simulink model "upravljani_nelinearni_i_linearni_model"  (R2015a)
settings: Solver=ode4  StartTime=0.0  StopTime=400  FixedStep=0.01  RelTol=1e-3
values from neighbouring files (symbols this model uses):
  a1 = K_dek(1, 1)    [skript_drugi_deo.m]
  a2 = K_dek(1, 2)    [skript_drugi_deo.m]
  a3 = K_dek(2, 1)    [skript_drugi_deo.m]
  a4 = K_dek(2, 2)    [skript_drugi_deo.m]
  Ar1 = 0.04    [skript_drugi_deo.m]
  Ar2 = 0.04    [skript_drugi_deo.m]
  Cd1 = 0.65    [skript_drugi_deo.m]
  Cd2 = 0.65    [skript_drugi_deo.m]
  Cdh = 0.65    [skript_drugi_deo.m]
  df1_H1 = double(subs(df1_H1, [Uvh Uv2 H1 H2], [Uvh_N Uv2_N H1_N H2_N]))    [skript_drugi_deo.m]
  df1_Uvh = double(subs(df1_Uvh, [Uvh Uv2 H1 H2], [Uvh_N Uv2_N H1_N H2_N]))    [skript_drugi_deo.m]
  df2_H1 = double(subs(df2_H1, [Uvh Uv2 H1 H2], [Uvh_N Uv2_N H1_N H2_N]))    [skript_drugi_deo.m]
  df2_H2 = double(subs(df2_H2, [Uvh Uv2 H1 H2], [Uvh_N Uv2_N H1_N H2_N]))    [skript_drugi_deo.m]
  df2_Uv2 = double(subs(df2_Uv2, [Uvh Uv2 H1 H2], [Uvh_N Uv2_N H1_N H2_N]))    [skript_drugi_deo.m]
  g = 9.81    [skript_drugi_deo.m]
  H1_max = 1.5    [skript_drugi_deo.m]
  H1_min = 0    [skript_drugi_deo.m]
  H1_N = 0.7    [skript_drugi_deo.m]
  H2_max = 1.5    [skript_drugi_deo.m]
  H2_min = 0    [skript_drugi_deo.m]
  H2_N = 0.8    [skript_drugi_deo.m]
  Kv1 = 1.5/1000    (= 0.0015)    [skript_drugi_deo.m]
  Kv2 = 1.5/1000    (= 0.0015)    [skript_drugi_deo.m]
  Kvh = 1/1000    (= 0.001)    [skript_drugi_deo.m]
  Ph = 3.25*10^5    (= 325000)    [skript_drugi_deo.m]
  ro = 1000    [skript_drugi_deo.m]
  Uv1 = 3    [skript_drugi_deo.m]
  Uv2_max = 10    [skript_drugi_deo.m]
  Uv2_min = 0    [skript_drugi_deo.m]
  Uv2_N = double(solve(e2 == 0, U2_N))    [skript_drugi_deo.m]
  Uvh_max = 10    [skript_drugi_deo.m]
  Uvh_min = 0    [skript_drugi_deo.m]
  Uvh_N = double(solve(e1 == 0, Uh_N))    [skript_drugi_deo.m]
  w1 = 0.1    [skript_drugi_deo.m]
  w2 = 0.1    [skript_drugi_deo.m]
  wh = 0.03    [skript_drugi_deo.m]
libraries: simulink x4
settings Model: Creator=Nikola  LastModifiedBy=Nikola

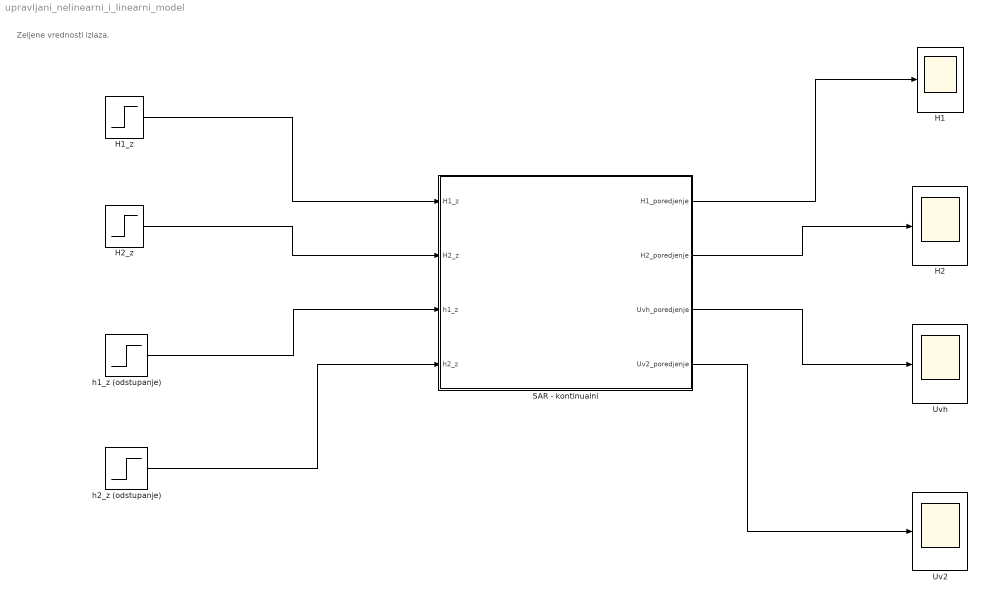
== system upravljani_nelinearni_i_linearni_model ==
  note: Zeljene vrednosti izlaza.
  " H2 " : Scope
      settings: SaveName=ScopeData4
  H1 : Scope
      settings: SaveName=ScopeData3
  "H1_z " : Step  Time=0  After=H1_N  SampleTime=0
  H2_z : Step  Time=0  After=H2_N  SampleTime=0
  SAR - kontinualni : Subsystem
  Uv2 : Scope
  "Uvh " : Scope
  h1_z (odstupanje) : Step  Time=0  After=0.1  SampleTime=0
  h2_z (odstupanje) : Step  Time=0  After=0  SampleTime=0
  wires:
  "H1_z "/1 -> SAR - kontinualni/1(H1_z)
  H2_z/1 -> SAR - kontinualni/2(H2_z)
  h1_z (odstupanje)/1 -> SAR - kontinualni/3(h1_z)
  h2_z (odstupanje)/1 -> SAR - kontinualni/4(h2_z)
  SAR - kontinualni/1(H1_poredjenje) -> H1/1
  SAR - kontinualni/2(H2_poredjenje) -> " H2 "/1
  SAR - kontinualni/3(Uvh_poredjenje) -> "Uvh "/1
  SAR - kontinualni/4(Uv2_poredjenje) -> Uv2/1

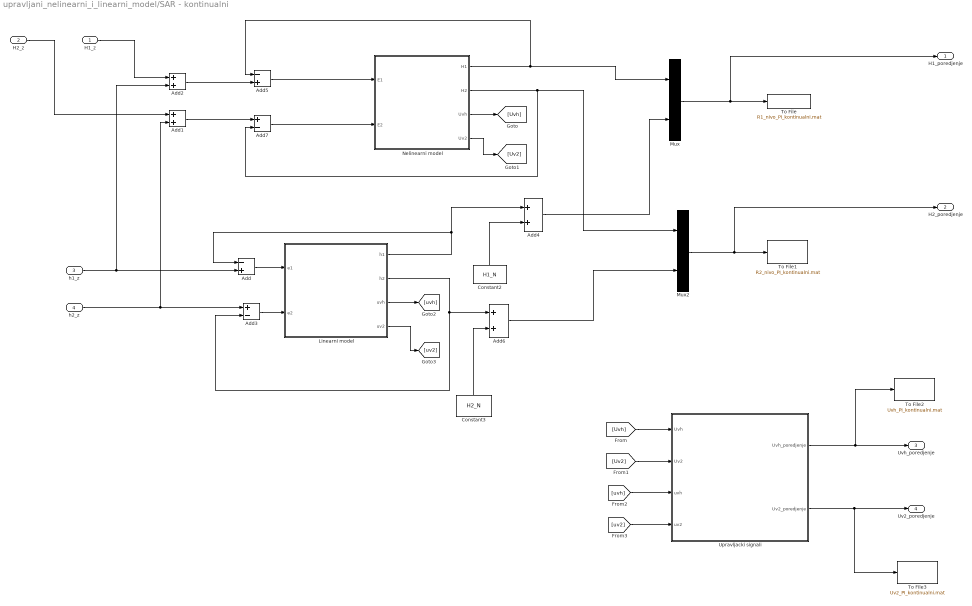
== system upravljani_nelinearni_i_linearni_model/SAR - kontinualni ==
  H1_z : Inport
  H2_z : Inport  Port=2
  h1_z : Inport  Port=3
  h2_z : Inport  Port=4
  Add : Sum  Inputs=-+
  Add{1..2,4,6} (4 alike) : Sum
  Add3 : Sum  Inputs=+-
  Add5 : Sum  Inputs=-+
  Add7 : Sum  Inputs=+-
  Constant2 : Constant  Value=H1_N
  Constant3 : Constant  Value=H2_N
  "Linearni model " : Subsystem
  Mux : Mux  Inputs=2
  Mux2 : Mux  Inputs=2
  "Nelinearni model " : Subsystem
  To File : ToFile  Filename=R1_nivo_PI_kontinualni.mat  MatrixName=H1_PI_kont
  To File1 : ToFile  Filename=R2_nivo_PI_kontinualni.mat  MatrixName=H2_PI_kont
  To File2 : ToFile  Filename=Uvh_PI_kontinualni.mat  MatrixName=Uvh_PI_kont
  To File3 : ToFile  Filename=Uv2_PI_kontinualni.mat  MatrixName=Uv2_PI_kont
  Upravljacki signali : Subsystem
  H1_poredjenje : Outport
  H2_poredjenje : Outport  Port=2
  Uvh_poredjenje : Outport  Port=3
  Uv2_poredjenje : Outport  Port=4
  wires:
  Mux/1 -> H1_poredjenje/1, To File/1
  Mux2/1 -> H2_poredjenje/1, To File1/1
  h1_z/1 -> Add2/2, Add/2
  h2_z/1 -> Add1/2, Add3/1
  Add4/1 -> Mux/2
  Add6/1 -> Mux2/2
  Constant3/1 -> Add6/2
  "Linearni model "/1(h1) -> Add4/1, Add/1
  "Linearni model "/2(h2) -> Add3/2, Add6/1
  Add/1 -> "Linearni model "/1(e1)
  Add3/1 -> "Linearni model "/2(e2)
  "Nelinearni model "/1(H1) -> Mux/1, Add5/1
  "Nelinearni model "/2(H2) -> Add7/2, Mux2/1
  Add2/1 -> Add5/2
  Add5/1 -> "Nelinearni model "/1(E1)
  Add7/1 -> "Nelinearni model "/2(E2)
  Add1/1 -> Add7/1
  Constant2/1 -> Add4/2
  "Nelinearni model "/3(Uvh) -> [Uvh]
  "Nelinearni model "/4(Uv2) -> [Uv2]
  "Linearni model "/3(uvh) -> [uvh]
  "Linearni model "/4(uv2) -> [uv2]
  H1_z/1 -> Add2/1
  H2_z/1 -> Add1/1
  [Uvh] -> Upravljacki signali/1(Uvh)
  [Uv2] -> Upravljacki signali/2(Uv2)
  Upravljacki signali/1(Uvh_poredjenje) -> To File2/1, Uvh_poredjenje/1
  Upravljacki signali/2(Uv2_poredjenje) -> To File3/1, Uv2_poredjenje/1
  [uvh] -> Upravljacki signali/3(uvh)
  [uv2] -> Upravljacki signali/4(uv2)

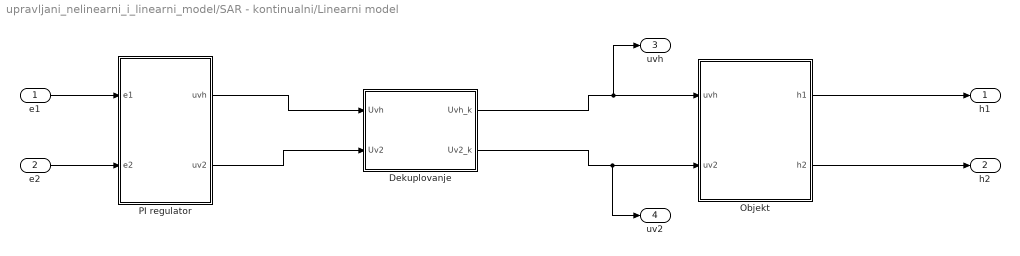
== system upravljani_nelinearni_i_linearni_model/SAR - kontinualni/Linearni model  ==
  e1 : Inport
  e2 : Inport  Port=2
  Dekuplovanje : Subsystem
  Objekt : Subsystem
  PI regulator : Subsystem
  h1 : Outport
  h2 : Outport  Port=2
  uvh : Outport  Port=3
  uv2 : Outport  Port=4
  wires:
  Objekt/1(h1) -> h1/1
  Objekt/2(h2) -> h2/1
  e1/1 -> PI regulator/1(e1)
  e2/1 -> PI regulator/2(e2)
  PI regulator/1(uvh) -> Dekuplovanje/1(Uvh)
  PI regulator/2(uv2) -> Dekuplovanje/2(Uv2)
  Dekuplovanje/1(Uvh_k) -> uvh/1, Objekt/1(uvh)
  Dekuplovanje/2(Uv2_k) -> uv2/1, Objekt/2(uv2)

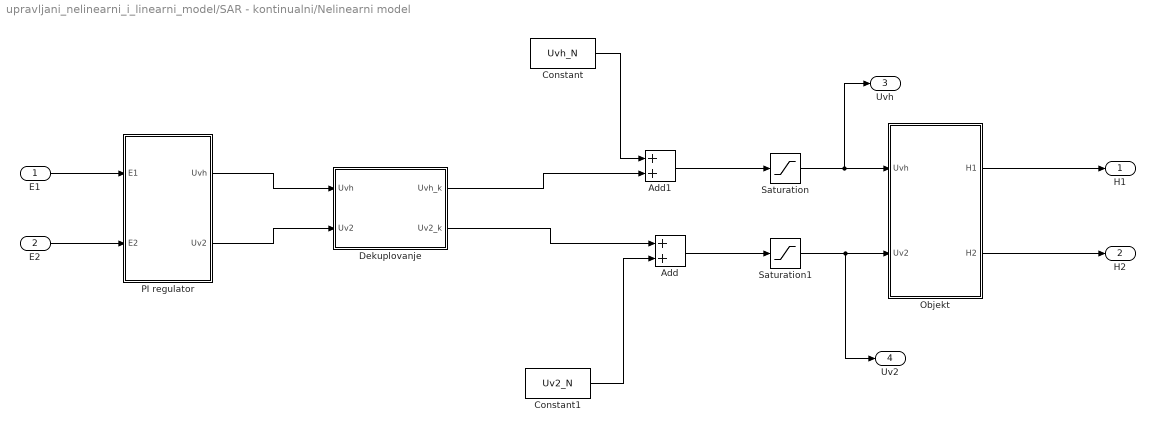
== system upravljani_nelinearni_i_linearni_model/SAR - kontinualni/Nelinearni model  ==
  E1 : Inport
  E2 : Inport  Port=2
  Add : Sum
  Add1 : Sum
  Constant : Constant  Value=Uvh_N
  Constant1 : Constant  Value=Uv2_N
  Dekuplovanje : Subsystem
  Objekt : Subsystem
  PI regulator : Subsystem
  Saturation : Saturate  UpperLimit=Uvh_max  LowerLimit=Uvh_min
  Saturation1 : Saturate  UpperLimit=Uv2_max  LowerLimit=Uv2_min
  H1 : Outport
  H2 : Outport  Port=2
  Uvh : Outport  Port=3
  Uv2 : Outport  Port=4
  wires:
  Objekt/1(H1) -> H1/1
  Objekt/2(H2) -> H2/1
  E2/1 -> PI regulator/2(E2)
  E1/1 -> PI regulator/1(E1)
  Saturation/1 -> Uvh/1, Objekt/1(Uvh)
  Saturation1/1 -> Uv2/1, Objekt/2(Uv2)
  Add1/1 -> Saturation/1
  Add/1 -> Saturation1/1
  Constant1/1 -> Add/2
  Constant/1 -> Add1/1
  Dekuplovanje/1(Uvh_k) -> Add1/2
  Dekuplovanje/2(Uv2_k) -> Add/1
  PI regulator/1(Uvh) -> Dekuplovanje/1(Uvh)
  PI regulator/2(Uv2) -> Dekuplovanje/2(Uv2)

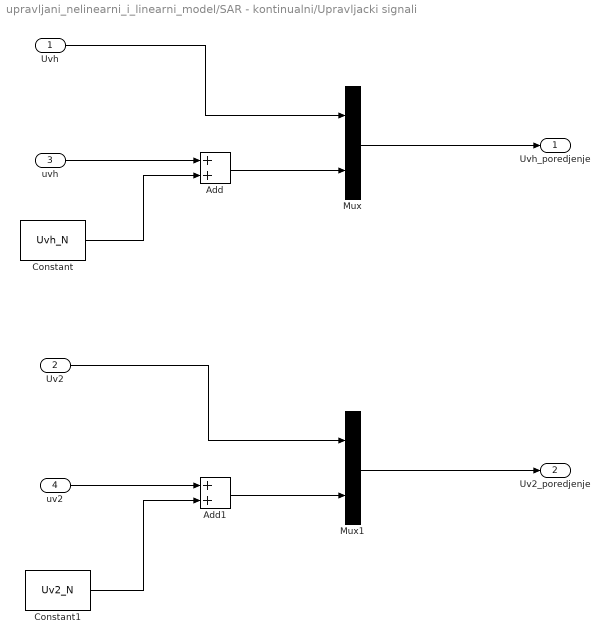
== system upravljani_nelinearni_i_linearni_model/SAR - kontinualni/Upravljacki signali ==
  Uvh : Inport
  Uv2 : Inport  Port=2
  uvh : Inport  Port=3
  uv2 : Inport  Port=4
  Add : Sum
  Add1 : Sum
  Constant : Constant  Value=Uvh_N
  Constant1 : Constant  Value=Uv2_N
  Mux : Mux  Inputs=2
  Mux1 : Mux  Inputs=2
  Uvh_poredjenje : Outport
  Uv2_poredjenje : Outport  Port=2
  wires:
  uvh/1 -> Add/1
  Constant/1 -> Add/2
  uv2/1 -> Add1/1
  Constant1/1 -> Add1/2
  Add/1 -> Mux/2
  Uvh/1 -> Mux/1
  Add1/1 -> Mux1/2
  Uv2/1 -> Mux1/1
  Mux/1 -> Uvh_poredjenje/1
  Mux1/1 -> Uv2_poredjenje/1

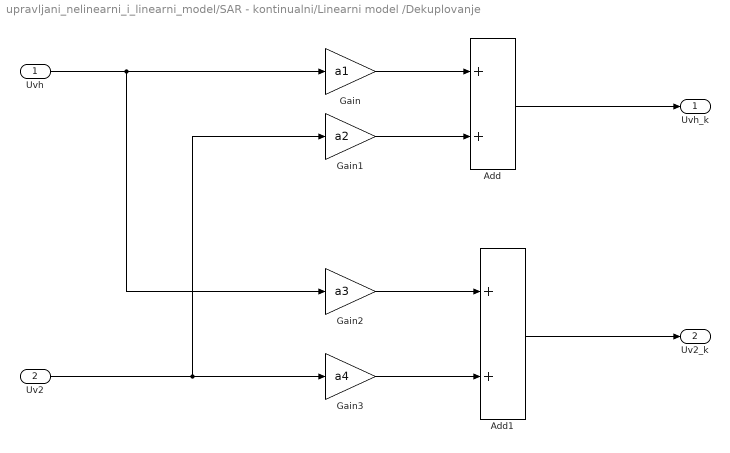
== system upravljani_nelinearni_i_linearni_model/SAR - kontinualni/Linearni model /Dekuplovanje ==
  Uvh : Inport
  Uv2 : Inport  Port=2
  Add : Sum
  Add1 : Sum
  Gain : Gain  Gain=a1
  Gain1 : Gain  Gain=a2
  Gain2 : Gain  Gain=a3
  Gain3 : Gain  Gain=a4
  Uvh_k : Outport
  Uv2_k : Outport  Port=2
  wires:
  Uvh/1 -> Gain2/1, Gain/1
  Uv2/1 -> Gain1/1, Gain3/1
  Gain/1 -> Add/1
  Gain1/1 -> Add/2
  Gain2/1 -> Add1/1
  Gain3/1 -> Add1/2
  Add/1 -> Uvh_k/1
  Add1/1 -> Uv2_k/1

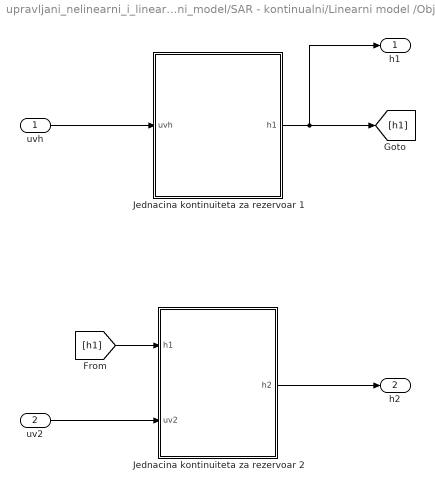
== system upravljani_nelinearni_i_linearni_model/SAR - kontinualni/Linearni model /Objekt ==
  uvh : Inport
  uv2 : Inport  Port=2
  Jednacina kontinuiteta za rezervoar 1 : Subsystem
  Jednacina kontinuiteta za rezervoar 2 : Subsystem
  h1 : Outport
  h2 : Outport  Port=2
  wires:
  Jednacina kontinuiteta za rezervoar 1/1(h1) -> [h1], h1/1
  [h1] -> Jednacina kontinuiteta za rezervoar 2/1(h1)
  Jednacina kontinuiteta za rezervoar 2/1(h2) -> h2/1
  uvh/1 -> Jednacina kontinuiteta za rezervoar 1/1(uvh)
  uv2/1 -> Jednacina kontinuiteta za rezervoar 2/2(uv2)

== system upravljani_nelinearni_i_linearni_model/SAR - kontinualni/Linearni model /PI regulator ==
  e1 : Inport
  e2 : Inport  Port=2
  PID Controller : simulink/Continuous/PID Controller  Controller=PI  TimeDomain=Continuous-time  SampleTime=-1  IntegratorMethod=Forward Euler  FilterMethod=Forward Euler  Form=Parallel  UseFilter=on  ControllerParametersSource=internal  P=6.58388823392313  I=0.318107260315565  D=0  N=100  InitialConditionSource=internal  InitialConditionForIntegrator=0  InitialConditionForFilter=0  ExternalReset=none  LimitOutput=off  UpperSaturationLimit=inf  LowerSaturationLimit=-inf  LinearizeAsGain=on  AntiWindupMode=none  Kb=1  TrackingMode=off  Kt=1  PParamMin=[]  PParamMax=[]  IParamMin=[]  IParamMax=[]  DParamMin=[]  DParamMax=[]  NParamMin=[]  NParamMax=[]  KbParamMin=[]  KbParamMax=[]  KtParamMin=[]  KtParamMax=[]  POutMin=[]  POutMax=[]  IOutMin=[]  IOutMax=[]  DOutMin=[]  DOutMax=[]  NOutMin=[]  NOutMax=[]  KbOutMin=[]  KbOutMax=[]  KtOutMin=[]  KtOutMax=[]  IntegratorOutMin=[]  IntegratorOutMax=[]  FilterOutMin=[]  FilterOutMax=[]  SumOutMin=[]  SumOutMax=[]  SumI1OutMin=[]  SumI1OutMax=[]  SumI2OutMin=[]  SumI2OutMax=[]  SumI3OutMin=[]  SumI3OutMax=[]  SumDOutMin=[]  SumDOutMax=[]  SaturationOutMin=[]  SaturationOutMax=[]  IntegratorContinuousStateAttributes=''  IntegratorStateMustResolveToSignalObject=off  IntegratorRTWStateStorageClass=Auto  FilterContinuousStateAttributes=''  FilterStateMustResolveToSignalObject=off  FilterRTWStateStorageClass=Auto  DifferentiatorICPrevScaledInput=0  DifferentiatorOutMin=[]  DifferentiatorOutMax=[]
  PID Controller1 : simulink/Continuous/PID Controller  Controller=PI  TimeDomain=Continuous-time  SampleTime=-1  IntegratorMethod=Forward Euler  FilterMethod=Forward Euler  Form=Parallel  UseFilter=on  ControllerParametersSource=internal  P=-9.63504962105945  I=-0.943120785670637  D=0  N=100  InitialConditionSource=internal  InitialConditionForIntegrator=0  InitialConditionForFilter=0  ExternalReset=none  LimitOutput=off  UpperSaturationLimit=inf  LowerSaturationLimit=-inf  LinearizeAsGain=on  AntiWindupMode=none  Kb=1  TrackingMode=off  Kt=1  PParamMin=[]  PParamMax=[]  IParamMin=[]  IParamMax=[]  DParamMin=[]  DParamMax=[]  NParamMin=[]  NParamMax=[]  KbParamMin=[]  KbParamMax=[]  KtParamMin=[]  KtParamMax=[]  POutMin=[]  POutMax=[]  IOutMin=[]  IOutMax=[]  DOutMin=[]  DOutMax=[]  NOutMin=[]  NOutMax=[]  KbOutMin=[]  KbOutMax=[]  KtOutMin=[]  KtOutMax=[]  IntegratorOutMin=[]  IntegratorOutMax=[]  FilterOutMin=[]  FilterOutMax=[]  SumOutMin=[]  SumOutMax=[]  SumI1OutMin=[]  SumI1OutMax=[]  SumI2OutMin=[]  SumI2OutMax=[]  SumI3OutMin=[]  SumI3OutMax=[]  SumDOutMin=[]  SumDOutMax=[]  SaturationOutMin=[]  SaturationOutMax=[]  IntegratorContinuousStateAttributes=''  IntegratorStateMustResolveToSignalObject=off  IntegratorRTWStateStorageClass=Auto  FilterContinuousStateAttributes=''  FilterStateMustResolveToSignalObject=off  FilterRTWStateStorageClass=Auto  DifferentiatorICPrevScaledInput=0  DifferentiatorOutMin=[]  DifferentiatorOutMax=[]
  uvh : Outport
  uv2 : Outport  Port=2
  wires:
  e1/1 -> PID Controller/1
  PID Controller/1 -> uvh/1
  e2/1 -> PID Controller1/1
  PID Controller1/1 -> uv2/1

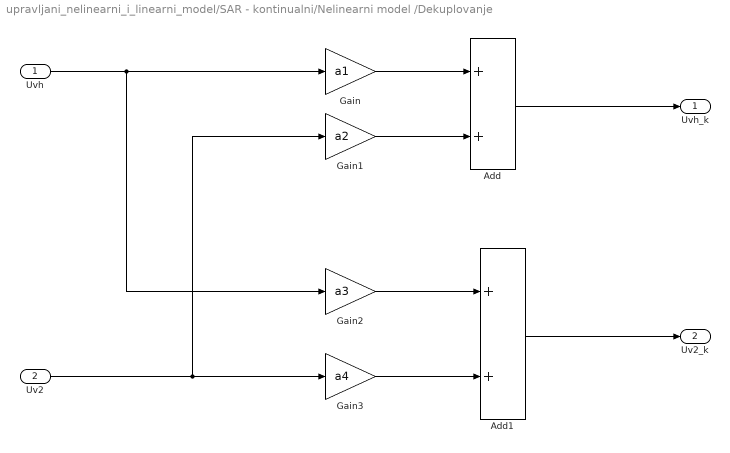
== system upravljani_nelinearni_i_linearni_model/SAR - kontinualni/Nelinearni model /Dekuplovanje ==
  Uvh : Inport
  Uv2 : Inport  Port=2
  Add : Sum
  Add1 : Sum
  Gain : Gain  Gain=a1
  Gain1 : Gain  Gain=a2
  Gain2 : Gain  Gain=a3
  Gain3 : Gain  Gain=a4
  Uvh_k : Outport
  Uv2_k : Outport  Port=2
  wires:
  Uvh/1 -> Gain2/1, Gain/1
  Uv2/1 -> Gain1/1, Gain3/1
  Gain/1 -> Add/1
  Gain1/1 -> Add/2
  Gain2/1 -> Add1/1
  Gain3/1 -> Add1/2
  Add/1 -> Uvh_k/1
  Add1/1 -> Uv2_k/1

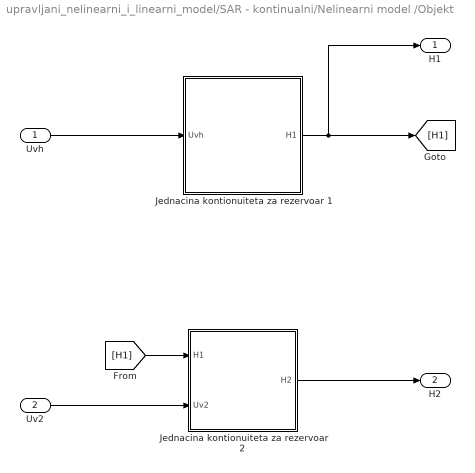
== system upravljani_nelinearni_i_linearni_model/SAR - kontinualni/Nelinearni model /Objekt ==
  Uvh : Inport
  Uv2 : Inport  Port=2
  Jednacina kontionuiteta za rezervoar 1 : Subsystem
  Jednacina kontionuiteta za rezervoar 2 : Subsystem
  H1 : Outport
  H2 : Outport  Port=2
  wires:
  Jednacina kontionuiteta za rezervoar 1/1(H1) -> [H1], H1/1
  Uvh/1 -> Jednacina kontionuiteta za rezervoar 1/1(Uvh)
  Uv2/1 -> Jednacina kontionuiteta za rezervoar 2/2(Uv2)
  Jednacina kontionuiteta za rezervoar 2/1(H2) -> H2/1
  [H1] -> Jednacina kontionuiteta za rezervoar 2/1(H1)

== system upravljani_nelinearni_i_linearni_model/SAR - kontinualni/Nelinearni model /PI regulator ==
  E1 : Inport
  E2 : Inport  Port=2
  PID Controller : simulink/Continuous/PID Controller  Controller=PI  TimeDomain=Continuous-time  SampleTime=-1  IntegratorMethod=Forward Euler  FilterMethod=Forward Euler  Form=Parallel  UseFilter=on  ControllerParametersSource=internal  P=6.58388823392313  I=0.318107260315565  D=0  N=100  InitialConditionSource=internal  InitialConditionForIntegrator=0  InitialConditionForFilter=0  ExternalReset=none  LimitOutput=off  UpperSaturationLimit=inf  LowerSaturationLimit=-inf  LinearizeAsGain=on  AntiWindupMode=none  Kb=1  TrackingMode=off  Kt=1  PParamMin=[]  PParamMax=[]  IParamMin=[]  IParamMax=[]  DParamMin=[]  DParamMax=[]  NParamMin=[]  NParamMax=[]  KbParamMin=[]  KbParamMax=[]  KtParamMin=[]  KtParamMax=[]  POutMin=[]  POutMax=[]  IOutMin=[]  IOutMax=[]  DOutMin=[]  DOutMax=[]  NOutMin=[]  NOutMax=[]  KbOutMin=[]  KbOutMax=[]  KtOutMin=[]  KtOutMax=[]  IntegratorOutMin=[]  IntegratorOutMax=[]  FilterOutMin=[]  FilterOutMax=[]  SumOutMin=[]  SumOutMax=[]  SumI1OutMin=[]  SumI1OutMax=[]  SumI2OutMin=[]  SumI2OutMax=[]  SumI3OutMin=[]  SumI3OutMax=[]  SumDOutMin=[]  SumDOutMax=[]  SaturationOutMin=[]  SaturationOutMax=[]  IntegratorContinuousStateAttributes=''  IntegratorStateMustResolveToSignalObject=off  IntegratorRTWStateStorageClass=Auto  FilterContinuousStateAttributes=''  FilterStateMustResolveToSignalObject=off  FilterRTWStateStorageClass=Auto  DifferentiatorICPrevScaledInput=0  DifferentiatorOutMin=[]  DifferentiatorOutMax=[]
  PID Controller2 : simulink/Continuous/PID Controller  Controller=PI  TimeDomain=Continuous-time  SampleTime=-1  IntegratorMethod=Forward Euler  FilterMethod=Forward Euler  Form=Parallel  UseFilter=on  ControllerParametersSource=internal  P=-9.63504962105945  I=-0.943120785670637  D=0  N=100  InitialConditionSource=internal  InitialConditionForIntegrator=0  InitialConditionForFilter=0  ExternalReset=none  LimitOutput=off  UpperSaturationLimit=inf  LowerSaturationLimit=-inf  LinearizeAsGain=on  AntiWindupMode=none  Kb=1  TrackingMode=off  Kt=1  PParamMin=[]  PParamMax=[]  IParamMin=[]  IParamMax=[]  DParamMin=[]  DParamMax=[]  NParamMin=[]  NParamMax=[]  KbParamMin=[]  KbParamMax=[]  KtParamMin=[]  KtParamMax=[]  POutMin=[]  POutMax=[]  IOutMin=[]  IOutMax=[]  DOutMin=[]  DOutMax=[]  NOutMin=[]  NOutMax=[]  KbOutMin=[]  KbOutMax=[]  KtOutMin=[]  KtOutMax=[]  IntegratorOutMin=[]  IntegratorOutMax=[]  FilterOutMin=[]  FilterOutMax=[]  SumOutMin=[]  SumOutMax=[]  SumI1OutMin=[]  SumI1OutMax=[]  SumI2OutMin=[]  SumI2OutMax=[]  SumI3OutMin=[]  SumI3OutMax=[]  SumDOutMin=[]  SumDOutMax=[]  SaturationOutMin=[]  SaturationOutMax=[]  IntegratorContinuousStateAttributes=''  IntegratorStateMustResolveToSignalObject=off  IntegratorRTWStateStorageClass=Auto  FilterContinuousStateAttributes=''  FilterStateMustResolveToSignalObject=off  FilterRTWStateStorageClass=Auto  DifferentiatorICPrevScaledInput=0  DifferentiatorOutMin=[]  DifferentiatorOutMax=[]
  Uvh : Outport
  Uv2 : Outport  Port=2
  wires:
  E1/1 -> PID Controller/1
  PID Controller/1 -> Uvh/1
  E2/1 -> PID Controller2/1
  PID Controller2/1 -> Uv2/1

== system upravljani_nelinearni_i_linearni_model/SAR - kontinualni/Linearni model /Objekt/Jednacina kontinuiteta za rezervoar 1 ==
  note: U sabiracu svugde stoji znak "+", umesto znaka "-", jer
      | su pojacanja dobijena u MATLAB-u sa
      | odgovarajucim predznakom.
  uvh : Inport
  Add : Sum
  Gain1 : Gain  Gain=df1_Uvh
  Gain3 : Gain  Gain=df1_H1
  Integrator : Integrator
  h1 : Outport
  wires:
  uvh/1 -> Gain1/1
  Add/1 -> Integrator/1  "dh1"
  Integrator/1 -> Gain3/1, h1/1  "h1"
  Gain3/1 -> Add/2
  Gain1/1 -> Add/1

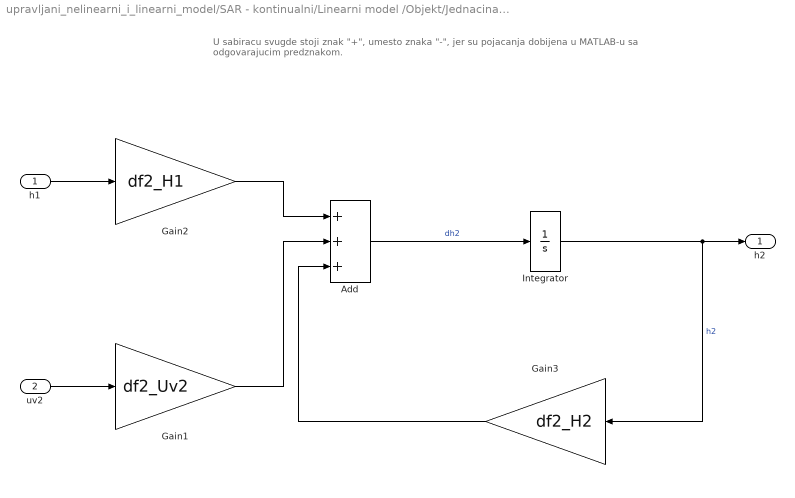
== system upravljani_nelinearni_i_linearni_model/SAR - kontinualni/Linearni model /Objekt/Jednacina kontinuiteta za rezervoar 2 ==
  note: U sabiracu svugde stoji znak "+", umesto znaka "-", jer
      | su pojacanja dobijena u MATLAB-u sa
      | odgovarajucim predznakom.
  h1 : Inport
  uv2 : Inport  Port=2
  Add : Sum  Inputs=+++
  Gain1 : Gain  Gain=df2_Uv2
  Gain2 : Gain  Gain=df2_H1
  Gain3 : Gain  Gain=df2_H2
  Integrator : Integrator
  h2 : Outport
  wires:
  Add/1 -> Integrator/1  "dh2"
  h1/1 -> Gain2/1
  Gain2/1 -> Add/1
  uv2/1 -> Gain1/1
  Gain1/1 -> Add/2
  Integrator/1 -> Gain3/1, h2/1  "h2"
  Gain3/1 -> Add/3

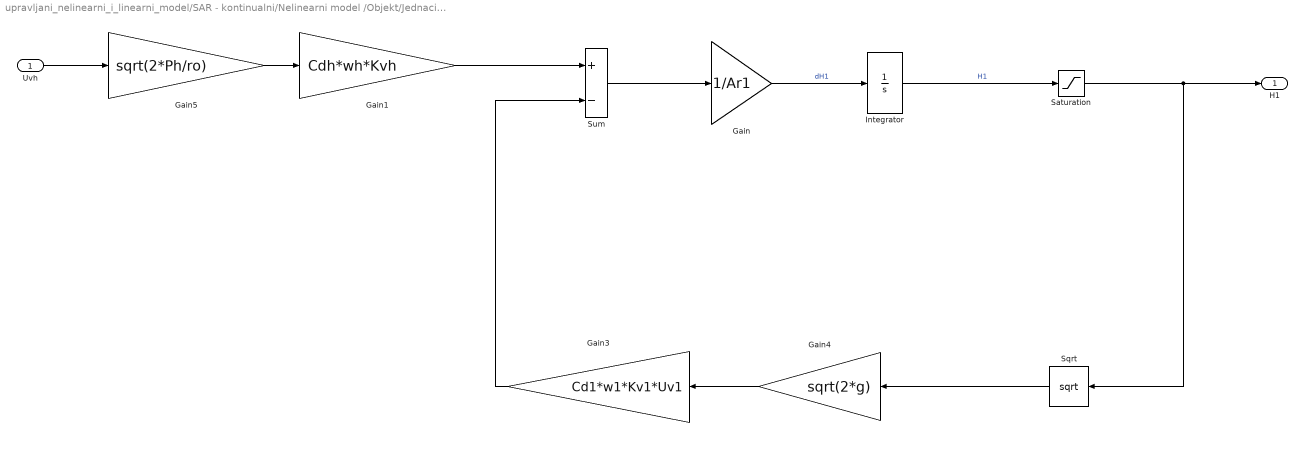
== system upravljani_nelinearni_i_linearni_model/SAR - kontinualni/Nelinearni model /Objekt/Jednacina kontionuiteta za rezervoar 1 ==
  Uvh : Inport
  Gain : Gain  Gain=1/Ar1
  Gain1 : Gain  Gain=Cdh*wh*Kvh
  Gain3 : Gain  Gain=Cd1*w1*Kv1*Uv1
  Gain4 : Gain  Gain=sqrt(2*g)
  Gain5 : Gain  Gain=sqrt(2*Ph/ro)
  Integrator : Integrator  InitialCondition=H1_N
  Saturation : Saturate  UpperLimit=H1_max  LowerLimit=H1_min
  Sqrt : Sqrt  SaturateOnIntegerOverflow=on
  Sum : Sum  Inputs=+-
  H1 : Outport
  wires:
  Gain/1 -> Integrator/1  "dH1"
  Sum/1 -> Gain/1
  Integrator/1 -> Saturation/1  "H1"
  Sqrt/1 -> Gain4/1
  Gain4/1 -> Gain3/1
  Gain5/1 -> Gain1/1
  Uvh/1 -> Gain5/1
  Saturation/1 -> Sqrt/1, H1/1
  Gain3/1 -> Sum/2
  Gain1/1 -> Sum/1

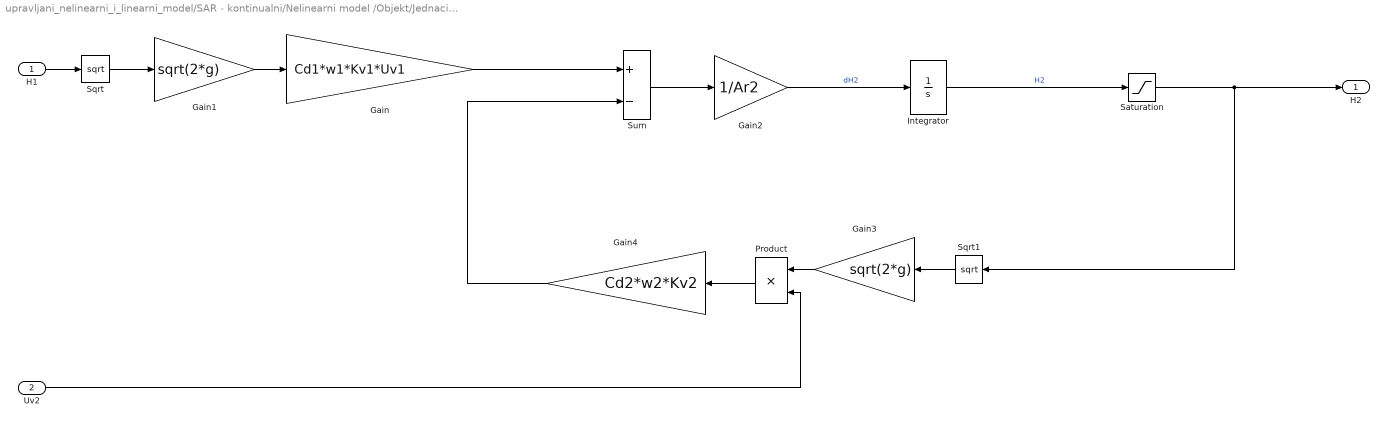
== system upravljani_nelinearni_i_linearni_model/SAR - kontinualni/Nelinearni model /Objekt/Jednacina kontionuiteta za rezervoar 2 ==
  H1 : Inport
  Uv2 : Inport  Port=2
  Gain : Gain  Gain=Cd1*w1*Kv1*Uv1
  Gain1 : Gain  Gain=sqrt(2*g)
  Gain2 : Gain  Gain=1/Ar2
  Gain3 : Gain  Gain=sqrt(2*g)
  Gain4 : Gain  Gain=Cd2*w2*Kv2
  Integrator : Integrator  InitialCondition=H2_N
  Product : Product
  Saturation : Saturate  UpperLimit=H2_max  LowerLimit=H2_min
  Sqrt : Sqrt  SaturateOnIntegerOverflow=on
  Sqrt1 : Sqrt  SaturateOnIntegerOverflow=on
  Sum : Sum  Inputs=+-
  H2 : Outport
  wires:
  H1/1 -> Sqrt/1
  Sqrt/1 -> Gain1/1
  Gain1/1 -> Gain/1
  Gain/1 -> Sum/1
  Sum/1 -> Gain2/1
  Gain2/1 -> Integrator/1  "dH2"
  Integrator/1 -> Saturation/1  "H2"
  Sqrt1/1 -> Gain3/1
  Gain3/1 -> Product/1
  Uv2/1 -> Product/2
  Product/1 -> Gain4/1
  Gain4/1 -> Sum/2
  Saturation/1 -> Sqrt1/1, H2/1
